simulink subsystem "LAB_01_19_SEPT_SIM_PENDOLO"  (R2022b)
settings: Solver=VariableStepAuto  StartTime=0.0  StopTime=10.0  RelTol=1e-3
values from neighbouring files (symbols this model uses):
  g = 9.81    [LAB_02_26_SEPT_MAT_PENDULUM.m]
  l = strcat([h,'',i])    [LAB_01_19_SEPT.m]    (also in LAB_02_26_SEPT_MAT_PENDULUM.m = 5)
settings Model: Creator=maria  LastModifiedBy=maria

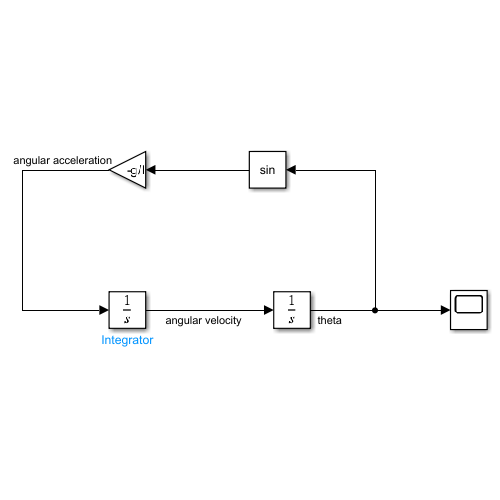
[thumbnail: Simulink's stored preview of the top-level diagram]
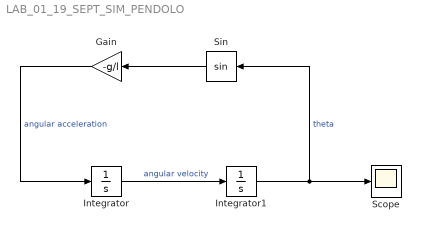
== system LAB_01_19_SEPT_SIM_PENDOLO ==
  Gain : Gain  Gain=-g/l
  Integrator : Integrator
  Integrator1 : Integrator  InitialCondition=1
  Scope : Scope
  Sin : Trigonometry
  wires:
  Integrator/1 -> Integrator1/1  "angular velocity"
  Sin/1 -> Gain/1
  Integrator1/1 -> Scope/1, Sin/1  "theta"
  Gain/1 -> Integrator/1  "angular acceleration"
